simulink model "controladores_carro_balanceo"  (R2019a)
settings: Solver=VariableStepAuto  StartTime=0.0  StopTime=120  RelTol=1e-3
InitFcn:
  | parametros
undefined symbols (not defined in the file): b_cx, b_cy, b_h_eq, b_hb, b_hEb, b_t, b_t_eq, b_tb, b_td_eq, b_tw, b_wu, g, H_c, i_h, i_t, K_cy, K_d_h, K_d_t, K_i_h, K_i_t, k_p3_th, K_p_h, K_p_t, k_th, K_tw, k_w_c_th, k_wu, l_h0, L_h0, M_c_max, M_c_min, m_h_eq, M_s, M_t, m_td_eq, overload, r_hd, r_td, sigbuilder_block, T_hb_max, T_hEb_max, T_hm_MAX, T_s2, T_tb_max, T_tm_max, tau_hm, tau_tm, v_h_max, W_c, w_hm_rated, x_l0, x_t0, x_t_max_emer, x_t_max_oper, x_t_min_emer, x_t_min_oper, x_td0, xi_c_th, y_h_max_emer, y_h_max_oper ... (+4)
libraries: simulink x10
(part 2 of 2)

== system controladores_carro_balanceo/Planta física/Izaje del carro/Modulador de torque en accionamiento de izaje/Reducción cuadrática de torque máximo (field weakening) ==
  note: Velocidad del motor de izaje
  note: Velocidad del motor de izaje equivalente
      | para velocidad de izaje nominal
  note: Torque de motor de izaje máximo
      | con reducción cuadrática
  note: Torque de motor de izaje máximo
      | para velocidades menores o igual
      | a la velocidad nominal del motor
  w_hm : Inport
  Constant1 : Constant  Value=w_hm_rated
  Constant2 : Constant
  Divide : Product  Inputs=*/  SaturateOnIntegerOverflow=on
  Gain : Gain  Gain=T_hm_MAX
  MinMax : MinMax  Inputs=2
  Square : Math  Operator=square  SaturateOnIntegerOverflow=on
  T_hm_max : Outport
  wires:
  Constant2/1 -> MinMax/1
  MinMax/1 -> Gain/1
  Gain/1 -> T_hm_max/1
  w_hm/1 -> Divide/2
  Constant1/1 -> Divide/1
  Divide/1 -> Square/1
  Square/1 -> MinMax/2

== system controladores_carro_balanceo/Planta física/Traslación del carro/Modulador de torque en accionamiento de carro/Limitador de torque máximo en tiempo discretizado ==
  note: Consigna de torque de motor de carro
  note: Consigna de torque de motor de carro
      | con limitación de torque máximo
  note: Modelo discretizado
      | k * T_s2 <= t < (k+1) * T_s2
  T_tm* : Inport
  Constant1 : Constant  Value=-T_tm_max
  Constant2 : Constant  Value=T_tm_max
  MinMax : MinMax  Inputs=2
  MinMax1 : MinMax  Function=max  Inputs=2
  Zero-Order Hold : ZeroOrderHold  SampleTime=T_s2
  Zero-Order Hold1 : ZeroOrderHold  SampleTime=T_s2
  T_tm_lim* : Outport
  wires:
  T_tm*/1 -> Zero-Order Hold/1
  MinMax/1 -> Zero-Order Hold1/1
  Constant1/1 -> MinMax1/1
  MinMax1/1 -> MinMax/2
  Zero-Order Hold/1 -> MinMax1/2
  Zero-Order Hold1/1 -> T_tm_lim*/1
  Constant2/1 -> MinMax/1

== matlab function controladores_carro_balanceo/Planta física/Carga suspendida/Perfil de obstáculos/MATLAB Function ==
  data: x_l input; y_c0_x_l output; TLK input; y_c0 output size=[1, 1651]; x_t_min_oper parameter double size=1; x_t_max_oper parameter double size=1; W_c parameter double size=1; H_c parameter double size=1; y_h_min_oper parameter double size=1
function [y_c0_x_l,y_c0] = update_perfil_obstactulos(x_l, TLK, x_t_min_oper, x_t_max_oper, W_c, H_c, y_h_min_oper)
    % Actualiza el perfil de obstaculos
    % Entradas:
    % 1) x_l: posición horizontal de la carga 
    % 2) TLK: twistlocks
    % Salidas:
    % 1) y_c0_x_l: perfil de obstáculo para la posición x_l y tiempo actual
    % 2) y_c0: perfil de obstáculo (vector de altura de obstáculos en
    % función de posición horizontal) para el tiempo actual
    
    persistent y_c0_prev x;

    if isempty(y_c0_prev)
        % Inicializar y_c0_prev si es la primera ejecución
        x_min = x_t_min_oper - W_c/2;
        x_max = x_t_max_oper + W_c/2;
        x = x_min:0.05:x_max; % Vector de posiciones horizontales
        y_c0_prev = y_h_min_oper * ones(1, size(x,2)); %Inicializa y_c0_prev con la posición vertical mínima
    end
    
    % Buscar índices donde x está en el rango [x_l ± H_c/2]
    indices = find((x >= (x_l - W_c/2)) & (x <= (x_l + W_c/2)));
    
    % Actualizar y_c0 para dichas posiciones.
    y_c0 = y_c0_prev; % Empieza con valores previos
    
    if (TLK)  % Si se abren los twistlocks (se suelta el contenedor)
        y_c0(indices) = y_c0(indices) + H_c;
    else      % Si se cierran los twistlocks (se agarra el contenedor)
        y_c0(indices) = y_c0(indices) - H_c;
    end
    
    % Buscar índice para x más cercano a x_l
    [~, index] = min(abs(x - x_l));
    y_c0_x_l = y_c0(index); % Actualiza valor de y_c0(x_l)
    
    % Guardar los valores actuales como previos para próxima iteración
    y_c0_prev = y_c0;
end

== matlab function controladores_carro_balanceo/Planta física/Carga suspendida/Parámetros de carga/Generate random load /MATLAB Function ==
  data: y output; min input; max input
function y = update_random(min, max)
    persistent r;
    if isempty(r)
        rng('shuffle'); % Shuffle the seed ONCE at the start
    end
    r = randi([min, max]); % Generate a new random integer on trigger
    y = r;
end

== matlab function controladores_carro_balanceo/Controladores de movimiento/Controlador de ángulo de balanceo/Des-linearización por retroalimentación/MATLAB Function ==
  data: theta input; a output; theta_dot input; x_t_dot input; l_h input; m_l input; g parameter double size=1; b_t_eq parameter double size=1; M_t parameter double size=1
function a = fcn(theta, theta_dot, x_t_dot, l_h, m_l, g, b_t_eq, M_t)
cos_theta = cos(theta);
sin_theta = sin(theta);

aux1 = m_l*g*sin_theta*cos_theta + m_l*l_h*sin_theta*theta_dot^2 - b_t_eq*x_t_dot;
aux2 = l_h*( M_t + m_l*sin_theta^2 );

a = -cos_theta * aux1 / aux2 - g*sin_theta/l_h;

== matlab function controladores_carro_balanceo/Controladores de movimiento/Controlador de ángulo de balanceo/Des-linearización por retroalimentación/MATLAB Function1 ==
  data: theta input; b output; l_h input; m_l input; M_t parameter double size=1
function b = fcn(theta, l_h, m_l, M_t)
cos_theta = cos(theta);
sin_theta = sin(theta);

b = -cos_theta / ( l_h*( M_t + m_l*sin_theta^2 ) );
